simulink model "HEV_Ctrl_V1"  (R2018a)
settings: Solver=FixedStepDiscrete  StartTime=0.0  StopTime=10.0  FixedStep=0.01  RelTol=1e-3  EnableMultiTasking=on
PreLoadFcn:
  | HEV_Ctrl_V1_PreLoad
undefined symbols (not defined in the file or in its folder): AstEnblEngSpdMin_H_K, AstEnblEngSpdMin_L_K, AstEnblSocMin_H_K, AstEnblSocMin_L_K, AstEnblVehSpdMin_H_K, AstEnblVehSpdMin_L_K, AstTrqCmpSOC_K2, AstTrqCmpSOC_X, AstTrqDstBase_K3, DifferentialGearRatio_K, DrvReqPropTrq_K3, DrvReqPropTrqMax_K, eHevCtrlMode, EngTrqMax_K2, EngTrqMax_K2x, HevCtrlEnbl_K, RchEnblEngSpdMin_H_K, RchEnblEngSpdMin_L_K, RchgEnblSocMax_H_K, RchgEnblSocMax_L_K, RchgTrqCmpSOC_K2, RchgTrqCmpSOC_X, RegnBrkCmpSOC_K2, RegnBrkCmpSOC_X, RegnBrkEnblBrkPdlMin_H_K, RegnBrkEnblBrkPdlMin_L_K, RegnBrkEnblSocMax_H_K, RegnBrkEnblSocMax_L_K, RegnBrkEnblVehSpdMin_H_K, RegnBrkEnblVehSpdMin_L_K, TransmissionGearRatio_K2
libraries: simulink x2
(part 2 of 2)

== system HEV_Ctrl_V1/Hev Control/Energy Management/DecideTransition/RegBrake/RS FlopFlop/if then elseif ==
  note: If then elseif
  if : Inport
  then1 : Inport  Port=2
  elseif : Inport  Port=3
  then2 : Inport  Port=4
  Data Type Conversion : DataTypeConversion  OutDataTypeStr=boolean
  Switch2 : Switch  Criteria=u2 ~= 0  Threshold=0.5  SaturateOnIntegerOverflow=on
      settings: AttributesFormatString=<%<Criteria>>
  Switch3 : Switch  Criteria=u2 ~= 0  Threshold=0.5  SaturateOnIntegerOverflow=on
      settings: AttributesFormatString=<%<Criteria>>
  Unit Delay : UnitDelay  SampleTime=-1
      settings: AttributesFormatString=<initial=%<X0>>\n<tsample=%<SampleTime>>
  y : Outport
  wires:
  then2/1 -> Switch2/1
  elseif/1 -> Switch2/2
  then1/1 -> Switch3/1
  Switch3/1 -> Unit Delay/1, Data Type Conversion/1  "y"
  Unit Delay/1 -> Switch2/3  "y_old"
  if/1 -> Switch3/2
  Switch2/1 -> Switch3/3
  Data Type Conversion/1 -> y/1

== stateflow chart HEV_Ctrl_V1/Hev Control/Energy Management/HevCtrlModeChart ==
  state HEV_control_mode
    state RegnBrake
      en:
      RegnBrk_event;
      HevCtrlMode = RegenBrake;
    state Assist
      en:
      Assist_event;
      HevCtrlMode = Assist;
    state ChargeBattery
      en:
      Rchg_event;
      HevCtrlMode = ReCharge;
    state EngineStart
      en:
      EngStart_event;
      HevCtrlMode = EngineStart;
    state MotorStandby
      en:
      Stby_event;
      HevCtrlMode = Standby;
    (default) -> (junction 3)
    HEV_control_mode -> (junction 3)
    (junction 3) -> RegnBrake [order 1] : [RegnBrkReq]
    (junction 3) -> (junction 9) [order 2]
    (junction 9) -> Assist [order 1] : [MtrAstReq]
    (junction 9) -> (junction 12) [order 2]
    (junction 12) -> ChargeBattery [order 1] : [RchgDrvReq]
    (junction 12) -> (junction 30) [order 2]
    (junction 30) -> EngineStart [order 1] : [EngStartReq]
    (junction 30) -> (junction 15) [order 2]
    (junction 15) -> MotorStandby
  data: RegnBrkReq input; HevCtrlMode output Enum: eHevCtrlMode; MtrAstReq input; RchgDrvReq input; EngStartReq input
  events: RegnBrk_event output FUNCTION_CALL_EVENT; Assist_event output FUNCTION_CALL_EVENT; Rchg_event output FUNCTION_CALL_EVENT; EngStart_event output FUNCTION_CALL_EVENT; Stby_event output FUNCTION_CALL_EVENT

== stateflow chart HEV_Ctrl_V1/Hev Control/Idle Stop/IdleStop_StateTransitionTable ==
  state IdleStop
    en:
    IdleStopCtrlMode=IdleStop;
  state EngineStart
    en:
    IdleStopCtrlMode=EngineStart;
  state IdleStopWait
  state IdleStopPrepare
    en:
    IdleStopCtrlMode=IdleStopWait;
  state EngineRun
    en:
    IdleStopCtrlMode=EngineRun;
  (default) -> IdleStop
  (junction 313) -> IdleStop
  IdleStop -> (junction 359) [order 2] : [EngSpd>300]%EngineRunCond
  (junction 350) -> (junction 313)
  (junction 359) -> (junction 355)
  IdleStop -> EngineStart [order 1] : [~IdleStopEnbl]%IdleStopEndCond
  EngineStart -> (junction 355) : [EngSpd>300]%EngineRunCond
  (junction 355) -> (junction 353)
  IdleStopWait -> (junction 350) : [EngSpd<50]%EngineStopCond
  (junction 339) -> (junction 350)
  IdleStopPrepare -> IdleStopWait [order 1] : [IdleStopEnbl]%IdleStopStartCond
  IdleStopPrepare -> (junction 339) [order 2] : [EngSpd<50]%EngineStopCond
  (junction 315) -> (junction 339)
  EngineRun -> IdleStopPrepare [order 1] : [IdleStopReq]%IdleStopWaitCond
  (junction 353) -> EngineRun
  EngineRun -> (junction 315) [order 2] : [EngSpd<50]%EngineStopCond
  data: IdleStopReq input; IdleStopEnbl input; EngSpd input; IdleStopCtrlMode output Enum: eIdleStopCtrlMode
